simulink model "slexPowerWindowCntlInteract"  (R2014b)
settings: Solver=ode23  StartTime=0  StopTime=10  FixedStep=1e-4  RelTol=1e-3
Description:
  | Interactively Test Controller
  | 
  | This model contains the power window controller which is a state
  | machine. This model also contains inputs to the controller which
  | are selected with manual switch blocks.
  | 
  | You can interactively test the controller by simulating the model
  | and selecting the desired combination of inputs via the manual
  | switch blocks.  After making the selection of inputs, you can verify
  | the internal controller state and controller output against the
  | desired result for this specific set of inputs.
settings Model: ExtModeAutoUpdateStatusClock=off  Creator=The MathWorks Inc.  LastModifiedBy=The MathWorks Inc.
settings DataIOCC: SignalLoggingName=sigsOut
settings OptimizationCC: ExpressionDepthLimit=2147483647
settings DebuggingCC: SaveWithParameterizedLinksMsg=none  UnderspecifiedInitializationDetection=Classic  MergeDetectMultiDrivingBlocksExec=none  SolverPrmCheckMsg=none  MultiTaskDSMMsg=warning  MultiTaskCondExecSysMsg=none  SigSpecEnsureSampleTimeMsg=none  FcnCallInpInsideContextMsg=UseLocalSettings  StateNameClashWarn=warning
settings HardwareCC: ProdHWDeviceType=Generic->Unspecified (assume 32-bit Generic)
settings SFSimCC: SimParseCustomCode=off
settings RTWCC: IncludeERTFirstTime=on
settings GRTTargetCC: TargetFcnLib=ansi_tfl_tmw.mat  CombineOutputUpdateFcns=off  GRTInterface=on

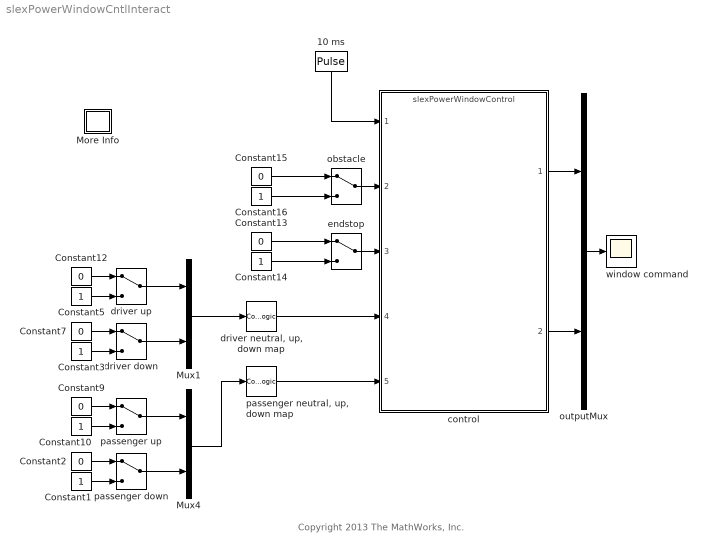
== system slexPowerWindowCntlInteract ==
  note: Copyright 2013 The MathWorks, Inc.
  10 ms : DiscretePulseGenerator  SampleTime=10e-3
  Constant{1,3,5,10,14,16} (6 alike) : Constant  OutDataTypeStr=boolean
  Constant{2,7,9,12..13,15} (6 alike) : Constant  Value=0  OutDataTypeStr=boolean
  More Info : Subsystem
      settings: OpenFcn=showdemo('slexPowerWindowScript')
      mask Display: disp('?')
  Mux1 : Mux  Inputs=2
  Mux4 : Mux  Inputs=2
  "control " : ModelReference  ModelNameDialog=slexPowerWindowControl.slx  SimulationMode=Normal  ModelReferenceVersion=1.83  CopyOfModelName=slexPowerWindowControl.slx  DefaultDataLogging=on
  "driver neutral, up, down map" : CombinatorialLogic  TruthTable=[1 0 0;0 0 1;0 1 0;1 0 0]
  driver down : ManualSwitch
  driver up : ManualSwitch
  endstop : ManualSwitch
  obstacle : ManualSwitch
  outputMux : Mux  Inputs=2
  "passenger neutral, up, down map" : CombinatorialLogic  TruthTable=[1 0 0;0 0 1;0 1 0;1 0 0]
  passenger down : ManualSwitch
  passenger up : ManualSwitch
  window command : Scope
      settings: YMin=0  YMax=1
  wires:
  Constant9/1 -> passenger up/1
  Constant10/1 -> passenger up/2
  Constant2/1 -> passenger down/1
  Constant1/1 -> passenger down/2
  passenger down/1 -> Mux4/2
  Constant12/1 -> driver up/1
  Constant5/1 -> driver up/2
  Constant7/1 -> driver down/1
  Constant3/1 -> driver down/2
  driver down/1 -> Mux1/2
  passenger up/1 -> Mux4/1
  driver up/1 -> Mux1/1
  "control "/1 -> outputMux/1
  "control "/2 -> outputMux/2
  outputMux/1 -> window command/1
  Mux4/1 -> "passenger neutral, up, down map"/1
  Mux1/1 -> "driver neutral, up, down map"/1
  "passenger neutral, up, down map"/1 -> "control "/5
  "driver neutral, up, down map"/1 -> "control "/4
  Constant13/1 -> endstop/1
  Constant14/1 -> endstop/2
  Constant15/1 -> obstacle/1
  Constant16/1 -> obstacle/2
  endstop/1 -> "control "/3
  obstacle/1 -> "control "/2
  10 ms/1 -> "control "/1

== system slexPowerWindowCntlInteract/More Info ==
